simulink model "SpeedControlTest_vDemo"  (Simulink 7.0)
settings: Solver=ode4  SolverMode=SingleTasking  StartTime=0.0  StopTime=252  FixedStep=0.01  RelTol=1e-3
InitFcn:
  | tempomat_para
StopFcn:
  | clear;
values from neighbouring files (symbols this model uses):
  A = 1.9    [tempomat_para.m]
  a_Fzg_max = 2    [tempomat_para.m]
  a_Fzg_min = -2    [tempomat_para.m]
  cw = 0.32    [tempomat_para.m]
  gang = [1 2 3 4]    [tempomat_para.m]
  gang_vec = [1 2 3 4]    [tempomat_para.m]
  i_anteil = 5    [tempomat_para.m]
  i_d = 3.42    [tempomat_para.m]
  i_g = [3.91 2.17 1.37 1.00]    [tempomat_para.m]
  lambda_gang = [1.3 1.25  1.17  1.05]    [tempomat_para.m]
  m_Fzg = 1400    [tempomat_para.m]
  M_mot_max = [130 149 163 170 168 166 162 158 150 139 123 80]    [tempomat_para.m]
  M_mot_min = [0 -40]    [tempomat_para.m]
  n_mot0 = 1000    [tempomat_para.m]
  n_mot_max = 1000:500:6500    [tempomat_para.m]
  n_mot_min = [1000 6500]    [tempomat_para.m]
  p_anteil = 100    [tempomat_para.m]
  r_dyn = 0.28    [tempomat_para.m]
  rho = 1.202    [tempomat_para.m]
  t_sch = 0.2    [tempomat_para.m]
  TI = [block '/TI']    [PSTI_callback.m]
  v_Fzg_ms0 = 0    [tempomat_para.m]
undefined symbols (not defined in the file or in its folder): Drossel_mat, getdatatypespecs
libraries: simulink x113, fzgbib x3
(part 9 of 10)

== system SpeedControlTest_vDemo/Validation Functions/R1 Speed Control step response/Maximum overshoot < 5 &  Steady state error < 5/Step response characteristics/Step response characteristics extraction/Extract maximum overshoot/Active if signals constant for some specified time ==
  Signal1 : Inport  OutDataType=sfix(16)  OutScaling=2^0
  Signal 2 : Inport  Port=2  OutDataType=sfix(16)  OutScaling=2^0
  Logical Operator1 : Logic  AllPortsSameDT=off  OutDataTypeMode=boolean
  Min Time : Constant  Value=5  OutDataType=sfix(16)  OutScaling=2^0
  MinMax : MinMax  Inputs=2  OutDataType=sfix(16)  OutScaling=2^0
  Relational Operator2 : RelationalOperator  Operator=<=  LogicOutDataTypeMode=boolean
  Switch : Switch  Criteria=u2 ~= 0
  Time since signal constant : Subsystem  TreatAsAtomicUnit=on  mask(Feature extraction block){RT=0.0001}
      mask prompts: RT "Relative tolerance in %"
      mask help: Detect if the signal value is constant (using the last two signal values) allowing for a user-defined relative deviation
      mask CallbackString:
      | if or( (str2double(get_param(gcb,'RT')) < 0), (str2double(get_param(gcb,'RT')) > 100))
      |     error(['Relative tolerance value (' get_param(gcb,'RT') ') out of range. Please give a value between 0 and 100.']);
      | else
      |     set_param([gcb '/Detect constant/Relative tolerance/Relative Tolerance'],'Value',get_param(gcb,'RT'));
      |     set_param([gcb '/Detect constant'],'RT',get_param(gcb,'RT'));
      | end
  Time since signal constant1 : Subsystem  TreatAsAtomicUnit=on  mask(Feature extraction block){RT=0.0001}
      mask prompts: RT "Relative tolerance in %"
      mask help: Detect if the signal value is constant (using the last two signal values) allowing for a user-defined relative deviation
      mask CallbackString:
      | if or( (str2double(get_param(gcb,'RT')) < 0), (str2double(get_param(gcb,'RT')) > 100))
      |     error(['Relative tolerance value (' get_param(gcb,'RT') ') out of range. Please give a value between 0 and 100.']);
      | else
      |     set_param([gcb '/Detect constant/Relative tolerance/Relative Tolerance'],'Value',get_param(gcb,'RT'));
      |     set_param([gcb '/Detect constant'],'RT',get_param(gcb,'RT'));
      | end
  Zero : Constant  Value=0  OutDataType=sfix(16)  OutScaling=2^0
  Constant signals : Outport  OutDataType=sfix(16)  OutScaling=2^0
  wires:
  Signal1/1 -> Time since signal constant/1(Signal)
  Signal 2/1 -> Time since signal constant1/1(Signal)
  Relational Operator2/1 -> Constant signals/1
  Min Time/1 -> Relational Operator2/1
  Switch/1 -> Relational Operator2/2
  Time since signal constant1/2(Feature) -> MinMax/2
  Time since signal constant/2(Feature) -> MinMax/1
  Time since signal constant/1(Trigger) -> Logical Operator1/1
  Time since signal constant1/1(Trigger) -> Logical Operator1/2
  MinMax/1 -> Switch/1
  Logical Operator1/1 -> Switch/2
  Zero/1 -> Switch/3

== system SpeedControlTest_vDemo/Validation Functions/R1 Speed Control step response/Maximum overshoot < 5 &  Steady state error < 5/Step response characteristics/Step response characteristics extraction/Extract maximum overshoot/Detect increase ==
  Signal : Inport  OutDataType=sfix(16)  OutScaling=2^0
  Clock : Clock
      settings: Decimation=10
  Memory : Memory
  Relational Operator : RelationalOperator  Operator=>  LogicOutDataTypeMode=Specify via dialog
  Switch : Switch  Criteria=u2 > Threshold
  Increase : Outport  OutDataType=sfix(16)  OutScaling=2^0
  wires:
  Switch/1 -> Relational Operator/2
  Memory/1 -> Switch/1
  Clock/1 -> Switch/2
  Relational Operator/1 -> Increase/1
  Signal/1 -> Switch/3, Memory/1, Relational Operator/1

== system SpeedControlTest_vDemo/Validation Functions/R1 Speed Control step response/Maximum overshoot < 5 &  Steady state error < 5/Step response characteristics/Step response characteristics extraction/Extract maximum overshoot/Detect increase1 ==
  Signal : Inport  OutDataType=sfix(16)  OutScaling=2^0
  Clock : Clock
      settings: Decimation=10
  Memory : Memory
  Relational Operator : RelationalOperator  Operator=>  LogicOutDataTypeMode=Specify via dialog
  Switch : Switch  Criteria=u2 > Threshold
  Increase : Outport  OutDataType=sfix(16)  OutScaling=2^0
  wires:
  Signal/1 -> Relational Operator/1, Memory/1, Switch/3
  Relational Operator/1 -> Increase/1
  Clock/1 -> Switch/2
  Memory/1 -> Switch/1
  Switch/1 -> Relational Operator/2

== system SpeedControlTest_vDemo/Validation Functions/R1 Speed Control step response/Maximum overshoot < 5 &  Steady state error < 5/Step response characteristics/Step response characteristics extraction/Extract maximum overshoot/Detect increase2 ==
  Signal : Inport  OutDataType=sfix(16)  OutScaling=2^0
  Clock : Clock
      settings: Decimation=10
  Memory : Memory
  Relational Operator : RelationalOperator  Operator=>  LogicOutDataTypeMode=Specify via dialog
  Switch : Switch  Criteria=u2 > Threshold
  Increase : Outport  OutDataType=sfix(16)  OutScaling=2^0
  wires:
  Switch/1 -> Relational Operator/2
  Memory/1 -> Switch/1
  Clock/1 -> Switch/2
  Relational Operator/1 -> Increase/1
  Signal/1 -> Switch/3, Memory/1, Relational Operator/1

== system SpeedControlTest_vDemo/Validation Functions/R1 Speed Control step response/Maximum overshoot < 5 &  Steady state error < 5/Step response characteristics/Step response characteristics extraction/Extract maximum overshoot/Hold value with counter ==
  Reset counter : Inport  OutDataType=sfix(16)  OutScaling=2^0
  Value : Inport  Port=2  OutDataType=sfix(16)  OutScaling=2^0
  Trigger : TriggerPort
  Execution counter : Subsystem  TreatAsAtomicUnit=on
  Memory : Memory  InheritSampleTime=on
  Number of executions : Constant  OutDataType=sfix(16)  OutScaling=2^0
  Relational Operator : RelationalOperator  Operator=<=  LogicOutDataTypeMode=boolean
  Switch : Switch  Criteria=u2 ~= 0
  Held value : Outport  OutDataType=sfix(16)  OutScaling=2^0
  wires:
  Memory/1 -> Switch/3
  Switch/1 -> Memory/1, Held value/1
  Value/1 -> Switch/1
  Reset counter/1 -> Execution counter/1(Reset)
  Number of executions/1 -> Relational Operator/2
  Execution counter/1(Counter) -> Relational Operator/1
  Relational Operator/1 -> Switch/2

== system SpeedControlTest_vDemo/Validation Functions/R1 Speed Control step response/Maximum overshoot < 5 &  Steady state error < 5/Step response characteristics/Step response characteristics extraction/Extract maximum overshoot/Step response moving average and initial conditions before step ==
  Reset : Inport  OutDataType=sfix(16)  OutScaling=2^0
  Step response : Inport  Port=2  OutDataType=sfix(16)  OutScaling=2^0
  Add2 : Sum  Inputs=+-  OutDataType=sfix(16)  OutScaling=2^-10
  Constant : Constant  Value=0  OutDataType=sfix(16)  OutScaling=2^0
  Flip if new step : Subsystem  TreatAsAtomicUnit=on
  Memory : Memory
  Switch : Switch  Criteria=u2 ~= 0
  Switch1 : Switch  Criteria=u2 ~= 0
  Switch2 : Switch  Criteria=u2 ~= 0
  Weighted Moving Average : S-Function  FunctionName=sfix_fir  Parameters=(getdatatypespecs(OutDataType,OutScaling,DblOver,0)),[DoSatur RndMeth-1],DblOver,dolog,mgainval,(getdatatypespecs(GainDataType,GainScaling,DblOver,RadixGroup)),samptime,vinit,OutputDataTypeScalingMode,GainDataTypeScalingMode  mask(Weighted Moving Average){mgainval=0.01*ones(1,100), vinit=0.0, samptime=-1, GainDataTypeScalingMode=Inherit via internal rule, GainDataType=sfix( 16 ), MatRadixGroup=Best Precision: Matrix-wise, GainScaling=2^-10, OutputDataTypeScalingMode=Inherit via internal rule, OutDataType=sfix(16), OutScaling=2^-10, LockScale=off, RndMeth=Floor, DoSatur=off}
      mask prompts: mgainval "Weights:"; vinit "Initial condition:"; samptime "Sample time:"; GainDataTypeScalingMode "Gain data type and scaling:"; GainDataType "Parameter data type:     ex. sfix(16),  uint(8), float('single')"; MatRadixGroup "Parameter scaling mode:"; GainScaling "Parameter scaling:    Slope    ex.  2^-9"; OutputDataTypeScalingMode "Output data type and scaling:"; OutDataType "Output data type:     ex.  sfix(16),  uint(8),  float('single')"; OutScaling "Output scaling:    Slope or [Slope Bias]    ex.  2^-9"; LockScale "Lock output scaling so autoscaling tool can't change it"; RndMeth "Round toward:"; DoSatur "Saturate to max or min when overflows occur"
      mask help: Output the weighted moving average of the input.
      mask init: same as SpeedControlTest_vDemo/Validation Functions/R1 Speed Control step response/Maximum overshoot < 5 &  Steady state error < 5/Step response characteristics/Step response characteristics extraction/Extract steady state error/Weighted Moving Average
      mask StyleString: edit,edit,edit,popup(Specify via dialog|Inherit via internal rule),edit,popup(Use Specified Scaling|Best Precision: Element-wise|Best Precision: Row-wise|Best Precision: Column-wise|Best Precision: Matrix-wise),edit,popup(Specify via dialog|Inherit via internal rule|Inherit via back propagation),edit,edit,checkbox,popup(Zero|Nearest|Ceiling|Floor),checkbox
      mask CallbackString: |||fixptdialog(gcbh)|fixptdialog(gcbh)|fixptdialog(gcbh)||fixptdialog(gcbh)|fixptdialog(gcbh)||||
      mask TabNameString: Main,Main,Main,Parameter data types,Parameter data types,Parameter data types,Parameter data types,Signal data types,Signal data types,Signal data types,Signal data types,Signal data types,Signal data types
      mask Display:
      | fprintf(fixpt_fir_mask_data(mgainval,'dispstr'))
      | plot(fixpt_fir_mask_data(mgainval,1),fixpt_fir_mask_data(mgainval,0))
  Weighted Moving Average1 : S-Function  FunctionName=sfix_fir  Parameters=(getdatatypespecs(OutDataType,OutScaling,DblOver,0)),[DoSatur RndMeth-1],DblOver,dolog,mgainval,(getdatatypespecs(GainDataType,GainScaling,DblOver,RadixGroup)),samptime,vinit,OutputDataTypeScalingMode,GainDataTypeScalingMode  mask(Weighted Moving Average){mgainval=0.01*ones(1,100), vinit=0.0, samptime=-1, GainDataTypeScalingMode=Inherit via internal rule, GainDataType=sfix( 16 ), MatRadixGroup=Best Precision: Matrix-wise, GainScaling=2^-10, OutputDataTypeScalingMode=Inherit via internal rule, OutDataType=sfix(16), OutScaling=2^-10, LockScale=off, RndMeth=Floor, DoSatur=off}
      mask prompts: mgainval "Weights:"; vinit "Initial condition:"; samptime "Sample time:"; GainDataTypeScalingMode "Gain data type and scaling:"; GainDataType "Parameter data type:     ex. sfix(16),  uint(8), float('single')"; MatRadixGroup "Parameter scaling mode:"; GainScaling "Parameter scaling:    Slope    ex.  2^-9"; OutputDataTypeScalingMode "Output data type and scaling:"; OutDataType "Output data type:     ex.  sfix(16),  uint(8),  float('single')"; OutScaling "Output scaling:    Slope or [Slope Bias]    ex.  2^-9"; LockScale "Lock output scaling so autoscaling tool can't change it"; RndMeth "Round toward:"; DoSatur "Saturate to max or min when overflows occur"
      mask help: Output the weighted moving average of the input.
      mask init: same as SpeedControlTest_vDemo/Validation Functions/R1 Speed Control step response/Maximum overshoot < 5 &  Steady state error < 5/Step response characteristics/Step response characteristics extraction/Extract steady state error/Weighted Moving Average
      mask StyleString: edit,edit,edit,popup(Specify via dialog|Inherit via internal rule),edit,popup(Use Specified Scaling|Best Precision: Element-wise|Best Precision: Row-wise|Best Precision: Column-wise|Best Precision: Matrix-wise),edit,popup(Specify via dialog|Inherit via internal rule|Inherit via back propagation),edit,edit,checkbox,popup(Zero|Nearest|Ceiling|Floor),checkbox
      mask CallbackString: |||fixptdialog(gcbh)|fixptdialog(gcbh)|fixptdialog(gcbh)||fixptdialog(gcbh)|fixptdialog(gcbh)||||
      mask TabNameString: Main,Main,Main,Parameter data types,Parameter data types,Parameter data types,Parameter data types,Signal data types,Signal data types,Signal data types,Signal data types,Signal data types,Signal data types
      mask Display:
      | fprintf(fixpt_fir_mask_data(mgainval,'dispstr'))
      | plot(fixpt_fir_mask_data(mgainval,1),fixpt_fir_mask_data(mgainval,0))
  d(Step Response) average : Outport  OutDataType=sfix(16)  OutScaling=2^0
  wires:
  Step response/1 -> Memory/1, Add2/1
  Memory/1 -> Add2/2
  Reset/1 -> Flip if new step/Enable
  Switch1/1 -> Weighted Moving Average/1
  Switch2/1 -> Weighted Moving Average1/1
  Weighted Moving Average/1 -> Switch/1
  Weighted Moving Average1/1 -> Switch/3
  Flip if new step/1(0/1) -> Switch1/2, Switch/2, Switch2/2
  Constant/1 -> Switch1/3, Switch2/1
  Add2/1 -> Switch2/3, Switch1/1
  Switch/1 -> d(Step Response) average/1

== system SpeedControlTest_vDemo/Validation Functions/R1 Speed Control step response/Maximum overshoot < 5 &  Steady state error < 5/Step response characteristics/Step response characteristics extraction/Extract maximum overshoot/Trigger hold value ==
  d(Step Response) average : Inport  OutDataType=sfix(16)  OutScaling=2^0
  Step sign : Inport  Port=2  OutDataType=sfix(16)  OutScaling=2^0
  Add : Sum  OutDataType=sfix(16)  OutScaling=2^-10
  Logical Operator1 : Logic  Operator=NOT  AllPortsSameDT=off  OutDataTypeMode=boolean
  Negative step : Subsystem  mask(Compare To Zero){relop=>, LogicOutDataTypeMode=uint8, ZeroCross=off}
      mask prompts: relop "Operator:"; LogicOutDataTypeMode "Output data type mode:"; ZeroCross "Enable zero crossing detection"
      mask help: Determine how a signal compares to zero.
      mask init:
      | blkName = gcb;
      | 
      | if strcmp(get_param(gcbh,'LogicOutDataTypeMode'),'boolean')
      | 	setValue = 'Boolean';
      | else
      |     setValue = 'Specify via dialog';
      | end
      | 
      | set_param([blkName,'/Compare'],'relop',relop, ...
      | 	'LogicOutDataTypeMode', setValue, 'ZeroCross', ZeroCross);
      mask StyleString: popup(==|~=|<|<=|>=|>),popup(uint8|boolean),checkbox
      mask Display: disp([relop,' 0'])
  Positive step : Subsystem  mask(Compare To Zero){relop=<, LogicOutDataTypeMode=uint8, ZeroCross=off}
      mask prompts: relop "Operator:"; LogicOutDataTypeMode "Output data type mode:"; ZeroCross "Enable zero crossing detection"
      mask help: Determine how a signal compares to zero.
      mask init: same as SpeedControlTest_vDemo/Validation Functions/R1 Speed Control step response/Maximum overshoot < 5 &  Steady state error < 5/Step response characteristics/Step response characteristics extraction/Extract maximum overshoot/Trigger hold value/Negative step
      mask StyleString: popup(==|~=|<|<=|>=|>),popup(uint8|boolean),checkbox
      mask Display: disp([relop,' 0'])
  Product : Product  OutDataType=sfix(16)  OutScaling=2^0  RndMeth=Zero
  Product1 : Product  OutDataType=sfix(16)  OutScaling=2^0  RndMeth=Zero
  Overshoot Trigger : Outport  OutDataType=sfix(16)  OutScaling=2^0
  wires:
  d(Step Response) average/1 -> Negative step/1(u), Positive step/1(u)
  Negative step/1(y) -> Product/1
  Positive step/1(y) -> Product1/2
  Step sign/1 -> Logical Operator1/1, Product1/1
  Product/1 -> Add/1
  Product1/1 -> Add/2
  Logical Operator1/1 -> Product/2
  Add/1 -> Overshoot Trigger/1

== system SpeedControlTest_vDemo/Validation Functions/R1 Speed Control step response/Maximum overshoot < 5 &  Steady state error < 5/Step response characteristics/Step response characteristics extraction/Extract rise time/Time difference ==
  Reset counter : Inport  OutDataType=sfix(16)  OutScaling=2^0
  Clock : Inport  Port=2  OutDataType=sfix(16)  OutScaling=2^0
  Trigger : TriggerPort  TriggerType=either
  Abs : Abs
  Execution counter : Subsystem  TreatAsAtomicUnit=on
  Memory : Memory  InheritSampleTime=on
  Memory1 : Memory  InheritSampleTime=on
  Number of executions : Constant  Value=3  OutDataType=sfix(16)  OutScaling=2^0
  Relational Operator : RelationalOperator  Operator=<=  LogicOutDataTypeMode=boolean
  Subtract : Sum  Inputs=+-  OutDataType=sfix(16)  OutScaling=2^-10
  Switch : Switch  Criteria=u2 ~= 0
  Time difference : Outport  OutDataType=sfix(16)  OutScaling=2^0
  wires:
  Clock/1 -> Switch/1
  Switch/1 -> Subtract/1, Memory/1
  Memory/1 -> Subtract/2, Memory1/1
  Memory1/1 -> Switch/3
  Relational Operator/1 -> Switch/2
  Subtract/1 -> Abs/1
  Abs/1 -> Time difference/1
  Number of executions/1 -> Relational Operator/2
  Reset counter/1 -> Execution counter/1(Reset)
  Execution counter/1(Counter) -> Relational Operator/1

== system SpeedControlTest_vDemo/Validation Functions/R1 Speed Control step response/Maximum overshoot < 5 &  Steady state error < 5/Step response characteristics/Step response characteristics extraction/Extract settling time/Time stamp ==
  Clock : Inport  OutDataType=sfix(16)  OutScaling=2^0
  Trigger : TriggerPort
  Time : Outport  OutDataType=sfix(16)  OutScaling=2^0
  wires:
  Clock/1 -> Time/1

== system SpeedControlTest_vDemo/Validation Functions/R1 Speed Control step response/Maximum overshoot < 5 &  Steady state error < 5/Step response characteristics/Step response reset/Active if signals constant for some specified time/Time since signal constant ==
  Signal : Inport  OutDataType=sfix(16)  OutScaling=2^0
  Clock : Clock
      settings: Decimation=10
  Detect constant : Subsystem  TreatAsAtomicUnit=on  mask(Feature extraction block){RT=0.0001}
      mask prompts: RT "Relative tolerance in %"
      mask help: Detect if the signal value is constant (using the last two signal values) allowing for a user-defined relative deviation
      mask CallbackString:
      | if or( (str2double(get_param(gcb,'RT')) < 0), (str2double(get_param(gcb,'RT')) > 100))
      |     error(['Relative tolerance value (' get_param(gcb,'RT') ') out of range. Please give a value between 0 and 100.']);
      | else
      |     set_param([gcb '/Relative tolerance/Relative Tolerance'],'Value',get_param(gcb,'RT'));
      | end
  Logical Operator : Logic  Operator=NAND  AllPortsSameDT=off  OutDataTypeMode=boolean
  Logical Operator1 : Logic  Operator=NOT  AllPortsSameDT=off  OutDataTypeMode=boolean
  Memory : Memory  Orientation=left
  Memory1 : Memory
  Subtract : Sum  Inputs=-+  OutDataType=sfix(16)  OutScaling=2^-10
  Switch : Switch  Criteria=u2 > Threshold
  Trigger : Outport  OutDataType=sfix(16)  OutScaling=2^0
  Feature : Outport  Port=2  OutDataType=sfix(16)  OutScaling=2^0
  wires:
  Signal/1 -> Detect constant/1(Signal)
  Detect constant/1(Constant) -> Trigger/1, Logical Operator/1, Memory1/1
  Subtract/1 -> Feature/1
  Clock/1 -> Subtract/2, Switch/3
  Switch/1 -> Subtract/1, Memory/1
  Memory/1 -> Switch/1
  Memory1/1 -> Logical Operator1/1
  Logical Operator1/1 -> Logical Operator/2
  Logical Operator/1 -> Switch/2

== system SpeedControlTest_vDemo/Validation Functions/R1 Speed Control step response/Maximum overshoot < 5 &  Steady state error < 5/Step response characteristics/Step response reset/Active if signals constant for some specified time/Time since signal constant1 ==
  Signal : Inport  OutDataType=sfix(16)  OutScaling=2^0
  Clock : Clock
      settings: Decimation=10
  Detect constant : Subsystem  TreatAsAtomicUnit=on  mask(Feature extraction block){RT=0.0001}
      mask prompts: RT "Relative tolerance in %"
      mask help: Detect if the signal value is constant (using the last two signal values) allowing for a user-defined relative deviation
      mask CallbackString:
      | if or( (str2double(get_param(gcb,'RT')) < 0), (str2double(get_param(gcb,'RT')) > 100))
      |     error(['Relative tolerance value (' get_param(gcb,'RT') ') out of range. Please give a value between 0 and 100.']);
      | else
      |     set_param([gcb '/Relative tolerance/Relative Tolerance'],'Value',get_param(gcb,'RT'));
      | end
  Logical Operator : Logic  Operator=NAND  AllPortsSameDT=off  OutDataTypeMode=boolean
  Logical Operator1 : Logic  Operator=NOT  AllPortsSameDT=off  OutDataTypeMode=boolean
  Memory : Memory  Orientation=left
  Memory1 : Memory
  Subtract : Sum  Inputs=-+  OutDataType=sfix(16)  OutScaling=2^-10
  Switch : Switch  Criteria=u2 > Threshold
  Trigger : Outport  OutDataType=sfix(16)  OutScaling=2^0
  Feature : Outport  Port=2  OutDataType=sfix(16)  OutScaling=2^0
  wires:
  Logical Operator/1 -> Switch/2
  Logical Operator1/1 -> Logical Operator/2
  Memory1/1 -> Logical Operator1/1
  Memory/1 -> Switch/1
  Switch/1 -> Memory/1, Subtract/1
  Clock/1 -> Switch/3, Subtract/2
  Subtract/1 -> Feature/1
  Detect constant/1(Constant) -> Memory1/1, Logical Operator/1, Trigger/1
  Signal/1 -> Detect constant/1(Signal)

== system SpeedControlTest_vDemo/Validation Functions/R1 Speed Control step response/Maximum overshoot < 5 &  Steady state error < 5/Step response characteristics/Step response trigger/Active if signals constant for some specified time/Time since signal constant ==
  Signal : Inport  OutDataType=sfix(16)  OutScaling=2^0
  Clock : Clock
      settings: Decimation=10
  Detect constant : Subsystem  TreatAsAtomicUnit=on  mask(Feature extraction block){RT=0.0001}
      mask prompts: RT "Relative tolerance in %"
      mask help: Detect if the signal value is constant (using the last two signal values) allowing for a user-defined relative deviation
      mask CallbackString:
      | if or( (str2double(get_param(gcb,'RT')) < 0), (str2double(get_param(gcb,'RT')) > 100))
      |     error(['Relative tolerance value (' get_param(gcb,'RT') ') out of range. Please give a value between 0 and 100.']);
      | else
      |     set_param([gcb '/Relative tolerance/Relative Tolerance'],'Value',get_param(gcb,'RT'));
      | end
  Logical Operator : Logic  Operator=NAND  AllPortsSameDT=off  OutDataTypeMode=boolean
  Logical Operator1 : Logic  Operator=NOT  AllPortsSameDT=off  OutDataTypeMode=boolean
  Memory : Memory  Orientation=left
  Memory1 : Memory
  Subtract : Sum  Inputs=-+  OutDataType=sfix(16)  OutScaling=2^-10
  Switch : Switch  Criteria=u2 > Threshold
  Trigger : Outport  OutDataType=sfix(16)  OutScaling=2^0
  Feature : Outport  Port=2  OutDataType=sfix(16)  OutScaling=2^0
  wires:
  Signal/1 -> Detect constant/1(Signal)
  Detect constant/1(Constant) -> Trigger/1, Logical Operator/1, Memory1/1
  Subtract/1 -> Feature/1
  Clock/1 -> Subtract/2, Switch/3
  Switch/1 -> Subtract/1, Memory/1
  Memory/1 -> Switch/1
  Memory1/1 -> Logical Operator1/1
  Logical Operator1/1 -> Logical Operator/2
  Logical Operator/1 -> Switch/2

== system SpeedControlTest_vDemo/Validation Functions/R1 Speed Control step response/Maximum overshoot < 5 &  Steady state error < 5/Step response characteristics/Step response trigger/Active if signals constant for some specified time/Time since signal constant1 ==
  Signal : Inport  OutDataType=sfix(16)  OutScaling=2^0
  Clock : Clock
      settings: Decimation=10
  Detect constant : Subsystem  TreatAsAtomicUnit=on  mask(Feature extraction block){RT=0.0001}
      mask prompts: RT "Relative tolerance in %"
      mask help: Detect if the signal value is constant (using the last two signal values) allowing for a user-defined relative deviation
      mask CallbackString:
      | if or( (str2double(get_param(gcb,'RT')) < 0), (str2double(get_param(gcb,'RT')) > 100))
      |     error(['Relative tolerance value (' get_param(gcb,'RT') ') out of range. Please give a value between 0 and 100.']);
      | else
      |     set_param([gcb '/Relative tolerance/Relative Tolerance'],'Value',get_param(gcb,'RT'));
      | end
  Logical Operator : Logic  Operator=NAND  AllPortsSameDT=off  OutDataTypeMode=boolean
  Logical Operator1 : Logic  Operator=NOT  AllPortsSameDT=off  OutDataTypeMode=boolean
  Memory : Memory  Orientation=left
  Memory1 : Memory
  Subtract : Sum  Inputs=-+  OutDataType=sfix(16)  OutScaling=2^-10
  Switch : Switch  Criteria=u2 > Threshold
  Trigger : Outport  OutDataType=sfix(16)  OutScaling=2^0
  Feature : Outport  Port=2  OutDataType=sfix(16)  OutScaling=2^0
  wires:
  Logical Operator/1 -> Switch/2
  Logical Operator1/1 -> Logical Operator/2
  Memory1/1 -> Logical Operator1/1
  Memory/1 -> Switch/1
  Switch/1 -> Memory/1, Subtract/1
  Clock/1 -> Switch/3, Subtract/2
  Subtract/1 -> Feature/1
  Detect constant/1(Constant) -> Memory1/1, Logical Operator/1, Trigger/1
  Signal/1 -> Detect constant/1(Signal)

== system SpeedControlTest_vDemo/Validation Functions/R2 Speed Control velocity restoration time after simple  acceleration or deceleration/CC active + no target & Speed Control active & step of V_Des = |1|  with time periods >= 7s/Step with step size=|1|  and time periods >= 6s detection/Step detection/Active if signals constant for some specified time/Time since signal constant1 ==
  Signal : Inport  OutDataType=sfix(16)  OutScaling=2^0
  Clock : Clock
      settings: Decimation=10
  Detect constant : Subsystem  TreatAsAtomicUnit=on  mask(Feature extraction block){RT=0.0001}
      mask prompts: RT "Relative tolerance in %"
      mask help: Detect if the signal value is constant (using the last two signal values) allowing for a user-defined relative deviation
      mask CallbackString:
      | if or( (str2double(get_param(gcb,'RT')) < 0), (str2double(get_param(gcb,'RT')) > 100))
      |     error(['Relative tolerance value (' get_param(gcb,'RT') ') out of range. Please give a value between 0 and 100.']);
      | else
      |     set_param([gcb '/Relative tolerance/Relative Tolerance'],'Value',get_param(gcb,'RT'));
      | end
  Logical Operator : Logic  Operator=NAND  AllPortsSameDT=off  OutDataTypeMode=boolean
  Logical Operator1 : Logic  Operator=NOT  AllPortsSameDT=off  OutDataTypeMode=boolean
  Memory : Memory  Orientation=left
  Memory1 : Memory
  Subtract : Sum  Inputs=-+  OutDataType=sfix(16)  OutScaling=2^-10
  Switch : Switch  Criteria=u2 > Threshold
  Trigger : Outport  OutDataType=sfix(16)  OutScaling=2^0
  Feature : Outport  Port=2  OutDataType=sfix(16)  OutScaling=2^0
  wires:
  Logical Operator/1 -> Switch/2
  Logical Operator1/1 -> Logical Operator/2
  Memory1/1 -> Logical Operator1/1
  Memory/1 -> Switch/1
  Switch/1 -> Memory/1, Subtract/1
  Clock/1 -> Switch/3, Subtract/2
  Subtract/1 -> Feature/1
  Detect constant/1(Constant) -> Memory1/1, Logical Operator/1, Trigger/1
  Signal/1 -> Detect constant/1(Signal)

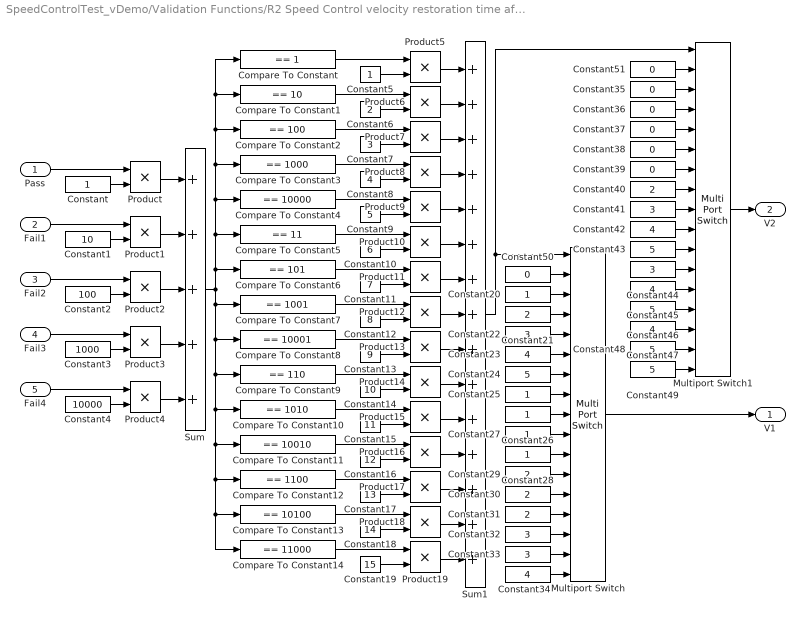
== system SpeedControlTest_vDemo/Validation Functions/R2 Speed Control velocity restoration time after simple  acceleration or deceleration/after (6 seconds)  |V_Des-V_Vhcl <= 1.4|/PAS1/none - pass - fail/Arbitration/Verdict identification ==
  Pass : Inport  OutDataType=sfix(16)  OutScaling=2^0
  Fail1 : Inport  Port=2  OutDataType=sfix(16)  OutScaling=2^0
  Fail2 : Inport  Port=3  OutDataType=sfix(16)  OutScaling=2^0
  Fail3 : Inport  Port=4  OutDataType=sfix(16)  OutScaling=2^0
  Fail4 : Inport  Port=5  OutDataType=sfix(16)  OutScaling=2^0
  Compare To Constant : simulink/Logic and Bit Operations/Compare To Constant  SystemSampleTime=-1  relop===  const=1  LogicOutDataTypeMode=uint8  ZeroCross=off
  Compare To Constant1 : simulink/Logic and Bit Operations/Compare To Constant  SystemSampleTime=-1  relop===  const=10  LogicOutDataTypeMode=uint8  ZeroCross=off
  Compare To Constant10 : simulink/Logic and Bit Operations/Compare To Constant  SystemSampleTime=-1  relop===  const=1010  LogicOutDataTypeMode=uint8  ZeroCross=off
  Compare To Constant11 : simulink/Logic and Bit Operations/Compare To Constant  SystemSampleTime=-1  relop===  const=10010  LogicOutDataTypeMode=uint8  ZeroCross=off
  Compare To Constant12 : simulink/Logic and Bit Operations/Compare To Constant  SystemSampleTime=-1  relop===  const=1100  LogicOutDataTypeMode=uint8  ZeroCross=off
  Compare To Constant13 : simulink/Logic and Bit Operations/Compare To Constant  SystemSampleTime=-1  relop===  const=10100  LogicOutDataTypeMode=uint8  ZeroCross=off
  Compare To Constant14 : simulink/Logic and Bit Operations/Compare To Constant  SystemSampleTime=-1  relop===  const=11000  LogicOutDataTypeMode=uint8  ZeroCross=off
  Compare To Constant2 : simulink/Logic and Bit Operations/Compare To Constant  SystemSampleTime=-1  relop===  const=100  LogicOutDataTypeMode=uint8  ZeroCross=off
  Compare To Constant3 : simulink/Logic and Bit Operations/Compare To Constant  SystemSampleTime=-1  relop===  const=1000  LogicOutDataTypeMode=uint8  ZeroCross=off
  Compare To Constant4 : simulink/Logic and Bit Operations/Compare To Constant  SystemSampleTime=-1  relop===  const=10000  LogicOutDataTypeMode=uint8  ZeroCross=off
  Compare To Constant5 : simulink/Logic and Bit Operations/Compare To Constant  SystemSampleTime=-1  relop===  const=11  LogicOutDataTypeMode=uint8  ZeroCross=off
  Compare To Constant6 : simulink/Logic and Bit Operations/Compare To Constant  SystemSampleTime=-1  relop===  const=101  LogicOutDataTypeMode=uint8  ZeroCross=off
  Compare To Constant7 : simulink/Logic and Bit Operations/Compare To Constant  SystemSampleTime=-1  relop===  const=1001  LogicOutDataTypeMode=uint8  ZeroCross=off
  Compare To Constant8 : simulink/Logic and Bit Operations/Compare To Constant  SystemSampleTime=-1  relop===  const=10001  LogicOutDataTypeMode=uint8  ZeroCross=off
  Compare To Constant9 : simulink/Logic and Bit Operations/Compare To Constant  SystemSampleTime=-1  relop===  const=110  LogicOutDataTypeMode=uint8  ZeroCross=off
  Constant{,5,20,25..28} (7 alike) : Constant  OutDataType=sfix(16)  OutScaling=2^0
  Constant1 : Constant  Value=10  OutDataType=sfix(16)  OutScaling=2^0
  Constant10 : Constant  Value=6  OutDataType=sfix(16)  OutScaling=2^0
  Constant11 : Constant  Value=7  OutDataType=sfix(16)  OutScaling=2^0
  Constant12 : Constant  Value=8  OutDataType=sfix(16)  OutScaling=2^0
  Constant13 : Constant  Value=9  OutDataType=sfix(16)  OutScaling=2^0
  Constant14 : Constant  Value=10  OutDataType=sfix(16)  OutScaling=2^0
  Constant15 : Constant  Value=11  OutDataType=sfix(16)  OutScaling=2^0
  Constant16 : Constant  Value=12  OutDataType=sfix(16)  OutScaling=2^0
  Constant17 : Constant  Value=13  OutDataType=sfix(16)  OutScaling=2^0
  Constant18 : Constant  Value=14  OutDataType=sfix(16)  OutScaling=2^0
  Constant19 : Constant  Value=15  OutDataType=sfix(16)  OutScaling=2^0
  Constant2 : Constant  Value=100  OutDataType=sfix(16)  OutScaling=2^0
  Constant{6,21,29..31,40} (6 alike) : Constant  Value=2  OutDataType=sfix(16)  OutScaling=2^0
  Constant{7,22,32..33,41,44} (6 alike) : Constant  Value=3  OutDataType=sfix(16)  OutScaling=2^0
  Constant{8,23,34,42,45,47} (6 alike) : Constant  Value=4  OutDataType=sfix(16)  OutScaling=2^0
  Constant{9,24,43,46,48..49} (6 alike) : Constant  Value=5  OutDataType=sfix(16)  OutScaling=2^0
  Constant3 : Constant  Value=1000  OutDataType=sfix(16)  OutScaling=2^0
  Constant{35..39,50..51} (7 alike) : Constant  Value=0  OutDataType=sfix(16)  OutScaling=2^0
  Constant4 : Constant  Value=10000  OutDataType=sfix(16)  OutScaling=2^0
  Multiport Switch : MultiPortSwitch  Inputs=16  zeroidx=on
  Multiport Switch1 : MultiPortSwitch  Inputs=16  zeroidx=on
  Product{,1..19} (20 alike) : Product  OutDataType=sfix(16)  OutScaling=2^0  RndMeth=Zero
  Sum : Sum  Inputs=+++++  OutDataType=sfix(16)  OutScaling=2^0
  Sum1 : Sum  Inputs=+++++++++++++++  OutDataType=sfix(16)  OutScaling=2^0
  V1 : Outport  OutDataType=sfix(16)  OutScaling=2^0
  V2 : Outport  Port=2  OutDataType=sfix(16)  OutScaling=2^0
  wires:
  Constant51/1 -> Multiport Switch1/2
  Constant34/1 -> Multiport Switch/17
  Constant33/1 -> Multiport Switch/16
  Constant32/1 -> Multiport Switch/15
  Constant31/1 -> Multiport Switch/14
  Constant30/1 -> Multiport Switch/13
  Constant29/1 -> Multiport Switch/12
  Constant28/1 -> Multiport Switch/11
  Constant27/1 -> Multiport Switch/10
  Constant26/1 -> Multiport Switch/9
  Constant25/1 -> Multiport Switch/8
  Constant24/1 -> Multiport Switch/7
  Constant23/1 -> Multiport Switch/6
  Constant22/1 -> Multiport Switch/5
  Constant21/1 -> Multiport Switch/4
  Constant20/1 -> Multiport Switch/3
  Constant50/1 -> Multiport Switch/2
  Product19/1 -> Sum1/15
  Product18/1 -> Sum1/14
  Product17/1 -> Sum1/13
  Product16/1 -> Sum1/12
  Product15/1 -> Sum1/11
  Product14/1 -> Sum1/10
  Product13/1 -> Sum1/9
  Product12/1 -> Sum1/8
  Product11/1 -> Sum1/7
  Product10/1 -> Sum1/6
  Product9/1 -> Sum1/5
  Product8/1 -> Sum1/4
  Product7/1 -> Sum1/3
  Product6/1 -> Sum1/2
  Product5/1 -> Sum1/1
  Multiport Switch1/1 -> V2/1
  Constant49/1 -> Multiport Switch1/17
  Constant48/1 -> Multiport Switch1/16
  Constant47/1 -> Multiport Switch1/15
  Constant46/1 -> Multiport Switch1/14
  Constant45/1 -> Multiport Switch1/13
  Constant44/1 -> Multiport Switch1/12
  Constant43/1 -> Multiport Switch1/11
  Constant42/1 -> Multiport Switch1/10
  Constant41/1 -> Multiport Switch1/9
  Constant40/1 -> Multiport Switch1/8
  Constant39/1 -> Multiport Switch1/7
  Constant38/1 -> Multiport Switch1/6
  Constant37/1 -> Multiport Switch1/5
  Constant36/1 -> Multiport Switch1/4
  Constant35/1 -> Multiport Switch1/3
  Sum1/1 -> Multiport Switch1/1, Multiport Switch/1
  Multiport Switch/1 -> V1/1
  Sum/1 -> Compare To Constant7/1, Compare To Constant13/1, Compare To Constant14/1, Compare To Constant12/1, Compare To Constant11/1, Compare To Constant10/1, Compare To Constant9/1, Compare To Constant8/1, Compare To Constant/1, Compare To Constant1/1, Compare To Constant2/1, Compare To Constant3/1, Compare To Constant4/1, Compare To Constant5/1, Compare To Constant6/1
  Compare To Constant14/1 -> Product19/1
  Constant19/1 -> Product19/2
  Compare To Constant13/1 -> Product18/1
  Constant18/1 -> Product18/2
  Compare To Constant12/1 -> Product17/1
  Constant17/1 -> Product17/2
  Compare To Constant11/1 -> Product16/1
  Constant16/1 -> Product16/2
  Compare To Constant10/1 -> Product15/1
  Constant15/1 -> Product15/2
  Compare To Constant9/1 -> Product14/1
  Constant14/1 -> Product14/2
  Compare To Constant8/1 -> Product13/1
  Constant13/1 -> Product13/2
  Compare To Constant7/1 -> Product12/1
  Constant12/1 -> Product12/2
  Compare To Constant6/1 -> Product11/1
  Constant11/1 -> Product11/2
  Compare To Constant5/1 -> Product10/1
  Constant10/1 -> Product10/2
  Compare To Constant4/1 -> Product9/1
  Constant9/1 -> Product9/2
  Compare To Constant3/1 -> Product8/1
  Compare To Constant2/1 -> Product7/1
  Constant8/1 -> Product8/2
  Constant7/1 -> Product7/2
  Compare To Constant1/1 -> Product6/1
  Constant6/1 -> Product6/2
  Constant5/1 -> Product5/2
  Compare To Constant/1 -> Product5/1
  Product4/1 -> Sum/5
  Product3/1 -> Sum/4
  Product2/1 -> Sum/3
  Product1/1 -> Sum/2
  Product/1 -> Sum/1
  Constant/1 -> Product/2
  Constant1/1 -> Product1/2
  Constant2/1 -> Product2/2
  Constant4/1 -> Product4/2
  Constant3/1 -> Product3/2
  Fail4/1 -> Product4/1
  Fail3/1 -> Product3/1
  Fail2/1 -> Product2/1
  Fail1/1 -> Product1/1
  Pass/1 -> Product/1

== system SpeedControlTest_vDemo/Validation Functions/R2 Speed Control velocity restoration time after simple  acceleration or deceleration/after (6 seconds)  |V_Des-V_Vhcl <= 1.4|/PAS1/none - pass - fail/Arbitration/Verdict selection ==
  V1 : Inport  OutDataType=sfix(16)  OutScaling=2^0
  V2 : Inport  Port=2  OutDataType=sfix(16)  OutScaling=2^0
  Delay P F1 F3 : Inport  Port=3  OutDataType=sfix(16)  OutScaling=2^0
  Delay F2 : Inport  Port=4  OutDataType=sfix(16)  OutScaling=2^0
  Delay F4 : Inport  Port=5  OutDataType=sfix(16)  OutScaling=2^0
  Max delay : Inport  Port=6  OutDataType=sfix(16)  OutScaling=2^0
  Compare To Zero1 : simulink/Logic and Bit Operations/Compare To Zero  SystemSampleTime=-1  relop=~=  LogicOutDataTypeMode=boolean  ZeroCross=off
  Constant{2..4,39} (4 alike) : Constant  Value=0  OutDataType=sfix(16)  OutScaling=2^0
  Constant35 : Constant  OutDataType=sfix(16)  OutScaling=2^0
  Constant40 : Constant  Value=2  OutDataType=sfix(16)  OutScaling=2^0
  Memory : Memory
  Memory1 : Memory
  Multiport Switch1 : MultiPortSwitch  Inputs=6  zeroidx=on
  Multiport Switch2 : MultiPortSwitch  Inputs=6  zeroidx=on
  Multiport Switch4 : MultiPortSwitch  Inputs=6  zeroidx=on
  Sum : Sum  OutDataType=sfix(16)  OutScaling=2^0
  Switch : Switch  Criteria=u2 ~= 0
  Switch1 : Switch  Criteria=u2 ~= 0
  Switch2 : Switch  Criteria=u2 ~= 0
  Unit : Constant  OutDataType=sfix(16)  OutScaling=2^0
  Verdict : Outport  OutDataType=sfix(16)  OutScaling=2^0
  Delay : Outport  Port=2  OutDataType=sfix(16)  OutScaling=2^0
  wires:
  Switch2/1 -> Multiport Switch4/1, Memory/1
  Unit/1 -> Sum/1
  Memory1/1 -> Sum/2
  Sum/1 -> Switch1/1
  Multiport Switch4/1 -> Memory1/1
  Multiport Switch2/1 -> Switch1/3
  Switch1/1 -> Delay/1
  Switch/1 -> Multiport Switch1/1
  Compare To Zero1/1 -> Switch2/2, Switch1/2, Switch/2
  Memory/1 -> Switch/1, Compare To Zero1/1
  Delay F4/1 -> Multiport Switch4/7, Multiport Switch2/7
  Delay F2/1 -> Multiport Switch4/5, Multiport Switch2/5
  Delay P F1 F3/1 -> Multiport Switch4/3, Multiport Switch4/4, Multiport Switch4/6, Multiport Switch2/4, Multiport Switch2/6, Multiport Switch2/3
  Max delay/1 -> Multiport Switch4/2, Multiport Switch2/2
  V1/1 -> Switch2/1, Switch/3, Multiport Switch2/1
  V2/1 -> Switch2/3
  Constant40/1 -> Multiport Switch1/2
  Constant35/1 -> Multiport Switch1/3
  Constant4/1 -> Multiport Switch1/4
  Constant3/1 -> Multiport Switch1/5
  Constant2/1 -> Multiport Switch1/6
  Constant39/1 -> Multiport Switch1/7
  Multiport Switch1/1 -> Verdict/1

== system SpeedControlTest_vDemo/Validation Functions/R2 Speed Control velocity restoration time after simple  acceleration or deceleration/after (6 seconds)  |V_Des-V_Vhcl <= 1.4|/PAS1/none - pass - fail/Compute delay/Hold1 ==
  " " : Inport  OutDataType=sfix(16)  OutScaling=2^0
  "    " : Inport  Port=2  OutDataType=sfix(16)  OutScaling=2^0
  Memory : Memory  Orientation=left
  Switch : Switch  Criteria=u2 ~= 0
  "  " : Outport  OutDataType=sfix(16)  OutScaling=2^0
  wires:
  " "/1 -> Switch/2
  "    "/1 -> Switch/1
  Switch/1 -> "  "/1, Memory/1
  Memory/1 -> Switch/3

== system SpeedControlTest_vDemo/Validation Functions/R2 Speed Control velocity restoration time after simple  acceleration or deceleration/after (6 seconds)  |V_Des-V_Vhcl <= 1.4|/PAS1/none - pass - fail/Compute delay1/Hold1 ==
  " " : Inport  OutDataType=sfix(16)  OutScaling=2^0
  "    " : Inport  Port=2  OutDataType=sfix(16)  OutScaling=2^0
  Memory : Memory  Orientation=left
  Switch : Switch  Criteria=u2 ~= 0
  "  " : Outport  OutDataType=sfix(16)  OutScaling=2^0
  wires:
  " "/1 -> Switch/2
  "    "/1 -> Switch/1
  Switch/1 -> "  "/1, Memory/1
  Memory/1 -> Switch/3

== system SpeedControlTest_vDemo/Validation Functions/R2 Speed Control velocity restoration time after simple  acceleration or deceleration/after (6 seconds)  |V_Des-V_Vhcl <= 1.4|/PAS1/none - pass - fail/Compute delay2/Hold1 ==
  " " : Inport  OutDataType=sfix(16)  OutScaling=2^0
  "    " : Inport  Port=2  OutDataType=sfix(16)  OutScaling=2^0
  Memory : Memory  Orientation=left
  Switch : Switch  Criteria=u2 ~= 0
  "  " : Outport  OutDataType=sfix(16)  OutScaling=2^0
  wires:
  Memory/1 -> Switch/3
  Switch/1 -> Memory/1, "  "/1
  "    "/1 -> Switch/1
  " "/1 -> Switch/2

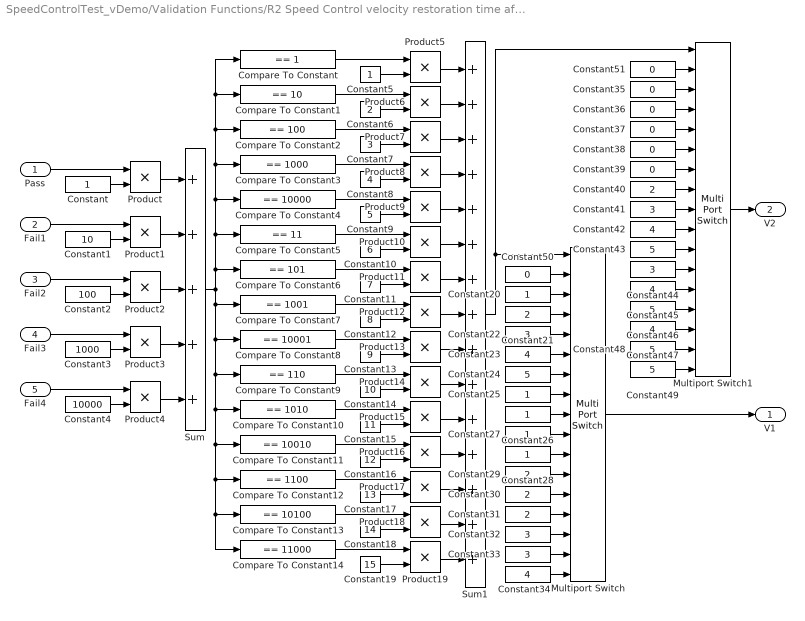
== system SpeedControlTest_vDemo/Validation Functions/R2 Speed Control velocity restoration time after simple  acceleration or deceleration/after (6 seconds)  |V_Des-V_Vhcl <= 1.4|/PAS2/none - pass - fail/Arbitration/Verdict identification ==
  Pass : Inport  OutDataType=sfix(16)  OutScaling=2^0
  Fail1 : Inport  Port=2  OutDataType=sfix(16)  OutScaling=2^0
  Fail2 : Inport  Port=3  OutDataType=sfix(16)  OutScaling=2^0
  Fail3 : Inport  Port=4  OutDataType=sfix(16)  OutScaling=2^0
  Fail4 : Inport  Port=5  OutDataType=sfix(16)  OutScaling=2^0
  Compare To Constant : simulink/Logic and Bit Operations/Compare To Constant  SystemSampleTime=-1  relop===  const=1  LogicOutDataTypeMode=uint8  ZeroCross=off
  Compare To Constant1 : simulink/Logic and Bit Operations/Compare To Constant  SystemSampleTime=-1  relop===  const=10  LogicOutDataTypeMode=uint8  ZeroCross=off
  Compare To Constant10 : simulink/Logic and Bit Operations/Compare To Constant  SystemSampleTime=-1  relop===  const=1010  LogicOutDataTypeMode=uint8  ZeroCross=off
  Compare To Constant11 : simulink/Logic and Bit Operations/Compare To Constant  SystemSampleTime=-1  relop===  const=10010  LogicOutDataTypeMode=uint8  ZeroCross=off
  Compare To Constant12 : simulink/Logic and Bit Operations/Compare To Constant  SystemSampleTime=-1  relop===  const=1100  LogicOutDataTypeMode=uint8  ZeroCross=off
  Compare To Constant13 : simulink/Logic and Bit Operations/Compare To Constant  SystemSampleTime=-1  relop===  const=10100  LogicOutDataTypeMode=uint8  ZeroCross=off
  Compare To Constant14 : simulink/Logic and Bit Operations/Compare To Constant  SystemSampleTime=-1  relop===  const=11000  LogicOutDataTypeMode=uint8  ZeroCross=off
  Compare To Constant2 : simulink/Logic and Bit Operations/Compare To Constant  SystemSampleTime=-1  relop===  const=100  LogicOutDataTypeMode=uint8  ZeroCross=off
  Compare To Constant3 : simulink/Logic and Bit Operations/Compare To Constant  SystemSampleTime=-1  relop===  const=1000  LogicOutDataTypeMode=uint8  ZeroCross=off
  Compare To Constant4 : simulink/Logic and Bit Operations/Compare To Constant  SystemSampleTime=-1  relop===  const=10000  LogicOutDataTypeMode=uint8  ZeroCross=off
  Compare To Constant5 : simulink/Logic and Bit Operations/Compare To Constant  SystemSampleTime=-1  relop===  const=11  LogicOutDataTypeMode=uint8  ZeroCross=off
  Compare To Constant6 : simulink/Logic and Bit Operations/Compare To Constant  SystemSampleTime=-1  relop===  const=101  LogicOutDataTypeMode=uint8  ZeroCross=off
  Compare To Constant7 : simulink/Logic and Bit Operations/Compare To Constant  SystemSampleTime=-1  relop===  const=1001  LogicOutDataTypeMode=uint8  ZeroCross=off
  Compare To Constant8 : simulink/Logic and Bit Operations/Compare To Constant  SystemSampleTime=-1  relop===  const=10001  LogicOutDataTypeMode=uint8  ZeroCross=off
  Compare To Constant9 : simulink/Logic and Bit Operations/Compare To Constant  SystemSampleTime=-1  relop===  const=110  LogicOutDataTypeMode=uint8  ZeroCross=off
  Constant{,5,20,25..28} (7 alike) : Constant  OutDataType=sfix(16)  OutScaling=2^0
  Constant1 : Constant  Value=10  OutDataType=sfix(16)  OutScaling=2^0
  Constant10 : Constant  Value=6  OutDataType=sfix(16)  OutScaling=2^0
  Constant11 : Constant  Value=7  OutDataType=sfix(16)  OutScaling=2^0
  Constant12 : Constant  Value=8  OutDataType=sfix(16)  OutScaling=2^0
  Constant13 : Constant  Value=9  OutDataType=sfix(16)  OutScaling=2^0
  Constant14 : Constant  Value=10  OutDataType=sfix(16)  OutScaling=2^0
  Constant15 : Constant  Value=11  OutDataType=sfix(16)  OutScaling=2^0
  Constant16 : Constant  Value=12  OutDataType=sfix(16)  OutScaling=2^0
  Constant17 : Constant  Value=13  OutDataType=sfix(16)  OutScaling=2^0
  Constant18 : Constant  Value=14  OutDataType=sfix(16)  OutScaling=2^0
  Constant19 : Constant  Value=15  OutDataType=sfix(16)  OutScaling=2^0
  Constant2 : Constant  Value=100  OutDataType=sfix(16)  OutScaling=2^0
  Constant{6,21,29..31,40} (6 alike) : Constant  Value=2  OutDataType=sfix(16)  OutScaling=2^0
  Constant{7,22,32..33,41,44} (6 alike) : Constant  Value=3  OutDataType=sfix(16)  OutScaling=2^0
  Constant{8,23,34,42,45,47} (6 alike) : Constant  Value=4  OutDataType=sfix(16)  OutScaling=2^0
  Constant{9,24,43,46,48..49} (6 alike) : Constant  Value=5  OutDataType=sfix(16)  OutScaling=2^0
  Constant3 : Constant  Value=1000  OutDataType=sfix(16)  OutScaling=2^0
  Constant{35..39,50..51} (7 alike) : Constant  Value=0  OutDataType=sfix(16)  OutScaling=2^0
  Constant4 : Constant  Value=10000  OutDataType=sfix(16)  OutScaling=2^0
  Multiport Switch : MultiPortSwitch  Inputs=16  zeroidx=on
  Multiport Switch1 : MultiPortSwitch  Inputs=16  zeroidx=on
  Product{,1..19} (20 alike) : Product  OutDataType=sfix(16)  OutScaling=2^0  RndMeth=Zero
  Sum : Sum  Inputs=+++++  OutDataType=sfix(16)  OutScaling=2^0
  Sum1 : Sum  Inputs=+++++++++++++++  OutDataType=sfix(16)  OutScaling=2^0
  V1 : Outport  OutDataType=sfix(16)  OutScaling=2^0
  V2 : Outport  Port=2  OutDataType=sfix(16)  OutScaling=2^0
  wires:
  Constant51/1 -> Multiport Switch1/2
  Constant34/1 -> Multiport Switch/17
  Constant33/1 -> Multiport Switch/16
  Constant32/1 -> Multiport Switch/15
  Constant31/1 -> Multiport Switch/14
  Constant30/1 -> Multiport Switch/13
  Constant29/1 -> Multiport Switch/12
  Constant28/1 -> Multiport Switch/11
  Constant27/1 -> Multiport Switch/10
  Constant26/1 -> Multiport Switch/9
  Constant25/1 -> Multiport Switch/8
  Constant24/1 -> Multiport Switch/7
  Constant23/1 -> Multiport Switch/6
  Constant22/1 -> Multiport Switch/5
  Constant21/1 -> Multiport Switch/4
  Constant20/1 -> Multiport Switch/3
  Constant50/1 -> Multiport Switch/2
  Product19/1 -> Sum1/15
  Product18/1 -> Sum1/14
  Product17/1 -> Sum1/13
  Product16/1 -> Sum1/12
  Product15/1 -> Sum1/11
  Product14/1 -> Sum1/10
  Product13/1 -> Sum1/9
  Product12/1 -> Sum1/8
  Product11/1 -> Sum1/7
  Product10/1 -> Sum1/6
  Product9/1 -> Sum1/5
  Product8/1 -> Sum1/4
  Product7/1 -> Sum1/3
  Product6/1 -> Sum1/2
  Product5/1 -> Sum1/1
  Multiport Switch1/1 -> V2/1
  Constant49/1 -> Multiport Switch1/17
  Constant48/1 -> Multiport Switch1/16
  Constant47/1 -> Multiport Switch1/15
  Constant46/1 -> Multiport Switch1/14
  Constant45/1 -> Multiport Switch1/13
  Constant44/1 -> Multiport Switch1/12
  Constant43/1 -> Multiport Switch1/11
  Constant42/1 -> Multiport Switch1/10
  Constant41/1 -> Multiport Switch1/9
  Constant40/1 -> Multiport Switch1/8
  Constant39/1 -> Multiport Switch1/7
  Constant38/1 -> Multiport Switch1/6
  Constant37/1 -> Multiport Switch1/5
  Constant36/1 -> Multiport Switch1/4
  Constant35/1 -> Multiport Switch1/3
  Sum1/1 -> Multiport Switch1/1, Multiport Switch/1
  Multiport Switch/1 -> V1/1
  Sum/1 -> Compare To Constant7/1, Compare To Constant13/1, Compare To Constant14/1, Compare To Constant12/1, Compare To Constant11/1, Compare To Constant10/1, Compare To Constant9/1, Compare To Constant8/1, Compare To Constant/1, Compare To Constant1/1, Compare To Constant2/1, Compare To Constant3/1, Compare To Constant4/1, Compare To Constant5/1, Compare To Constant6/1
  Compare To Constant14/1 -> Product19/1
  Constant19/1 -> Product19/2
  Compare To Constant13/1 -> Product18/1
  Constant18/1 -> Product18/2
  Compare To Constant12/1 -> Product17/1
  Constant17/1 -> Product17/2
  Compare To Constant11/1 -> Product16/1
  Constant16/1 -> Product16/2
  Compare To Constant10/1 -> Product15/1
  Constant15/1 -> Product15/2
  Compare To Constant9/1 -> Product14/1
  Constant14/1 -> Product14/2
  Compare To Constant8/1 -> Product13/1
  Constant13/1 -> Product13/2
  Compare To Constant7/1 -> Product12/1
  Constant12/1 -> Product12/2
  Compare To Constant6/1 -> Product11/1
  Constant11/1 -> Product11/2
  Compare To Constant5/1 -> Product10/1
  Constant10/1 -> Product10/2
  Compare To Constant4/1 -> Product9/1
  Constant9/1 -> Product9/2
  Compare To Constant3/1 -> Product8/1
  Compare To Constant2/1 -> Product7/1
  Constant8/1 -> Product8/2
  Constant7/1 -> Product7/2
  Compare To Constant1/1 -> Product6/1
  Constant6/1 -> Product6/2
  Constant5/1 -> Product5/2
  Compare To Constant/1 -> Product5/1
  Product4/1 -> Sum/5
  Product3/1 -> Sum/4
  Product2/1 -> Sum/3
  Product1/1 -> Sum/2
  Product/1 -> Sum/1
  Constant/1 -> Product/2
  Constant1/1 -> Product1/2
  Constant2/1 -> Product2/2
  Constant4/1 -> Product4/2
  Constant3/1 -> Product3/2
  Fail4/1 -> Product4/1
  Fail3/1 -> Product3/1
  Fail2/1 -> Product2/1
  Fail1/1 -> Product1/1
  Pass/1 -> Product/1
